simulink model "Roteiro1"  (R2015a)
settings: Solver=ode45  StartTime=0.0  StopTime=3  RelTol=1e-3
undefined symbols (not defined in the file): G1
settings Model: Creator=Aluno  LastModifiedBy=Aluno

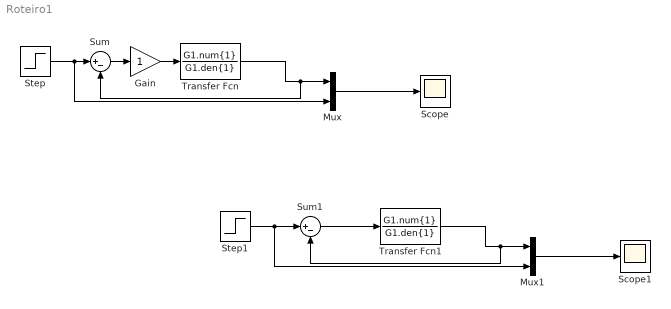
== system Roteiro1 ==
  Gain : Gain
  Mux : Mux  Inputs=2
  Mux1 : Mux  Inputs=2
  Scope : Scope
  Scope1 : Scope
  Step : Step  SampleTime=0
  Step1 : Step  SampleTime=0
  Sum : Sum  Inputs=|+-
  Sum1 : Sum  Inputs=|+-
  Transfer Fcn : TransferFcn  Numerator=G1.num{1}  Denominator=G1.den{1}
  Transfer Fcn1 : TransferFcn  Numerator=G1.num{1}  Denominator=G1.den{1}
  wires:
  Step/1 -> Sum/1, Mux/2
  Mux/1 -> Scope/1
  Transfer Fcn/1 -> Sum/2, Mux/1
  Step1/1 -> Mux1/2, Sum1/1
  Mux1/1 -> Scope1/1
  Transfer Fcn1/1 -> Sum1/2, Mux1/1
  Sum1/1 -> Transfer Fcn1/1
  Sum/1 -> Gain/1
  Gain/1 -> Transfer Fcn/1
